simulink model "tf_rl_reward2"  (R2022a)
settings: Solver=VariableStepAuto  StartTime=0.0  StopTime=10.0  RelTol=1e-3
undefined symbols (not defined in the file or in its folder): DiscIntNeverNeededParam
libraries: simulink x3, rllib x1
settings Model: Creator=vicky  LastModifiedBy=archi

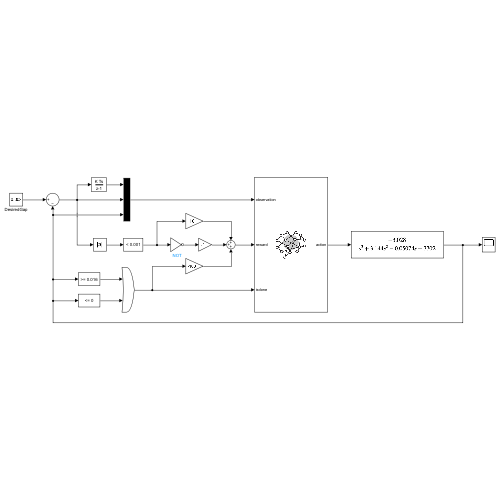
[thumbnail: Simulink's stored preview of the top-level diagram]
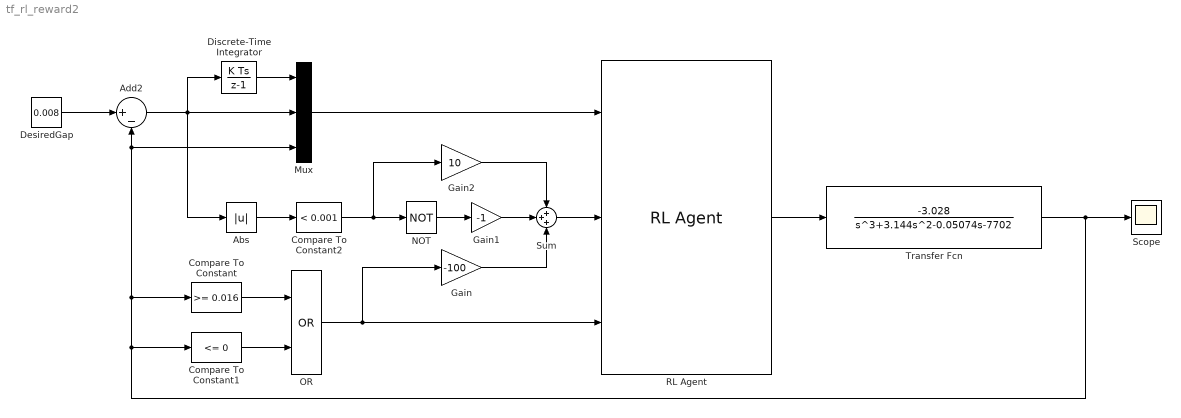
== system tf_rl_reward2 ==
  Abs : Abs  SaturateOnIntegerOverflow=off
  Add2 : Sum  Inputs=|+-
  Compare To Constant : simulink/Logic and Bit Operations/Compare To Constant  relop=>=  const=0.016  OutDataTypeStr=boolean
  Compare To Constant1 : simulink/Logic and Bit Operations/Compare To Constant  relop=<=  const=0  OutDataTypeStr=boolean
  Compare To Constant2 : simulink/Logic and Bit Operations/Compare To Constant  relop=<  const=0.001  OutDataTypeStr=boolean
  DesiredGap : Constant  Value=0.008
  Discrete-Time Integrator : DiscreteIntegrator  SampleTime=-1  ICPrevOutput=DiscIntNeverNeededParam  ICPrevScaledInput=DiscIntNeverNeededParam
  Gain : Gain  Gain=-100
  Gain1 : Gain  Gain=-1
  Gain2 : Gain  Gain=10
  Mux : Mux  Inputs=3
  NOT : Logic  Operator=NOT  IconShape=distinctive  AllPortsSameDT=off  OutDataTypeStr=boolean
  OR : Logic  Operator=OR  IconShape=distinctive  AllPortsSameDT=off  OutDataTypeStr=boolean
  RL Agent : rllib/RL Agent  Agent=rlDDPGAgent  ExternalActionAsInput=off  ProvideLastAction=off  ProvideCumRwd=off  TreatAsDirectFeedthrough=on  UseStrictObservationDataTypes=off
  Scope : Scope
  Sum : Sum  Inputs=+++
  Transfer Fcn : TransferFcn  Numerator=[-3.028]  Denominator=[1 3.144 -0.05074 -7702]
  wires:
  RL Agent/1 -> Transfer Fcn/1
  Add2/1 -> Mux/2, Abs/1, Discrete-Time Integrator/1
  Discrete-Time Integrator/1 -> Mux/1
  Mux/1 -> RL Agent/1
  DesiredGap/1 -> Add2/1
  Compare To Constant/1 -> OR/1
  Compare To Constant1/1 -> OR/2
  OR/1 -> Gain/1, RL Agent/3
  Transfer Fcn/1 -> Scope/1, Compare To Constant1/1, Compare To Constant/1, Mux/3, Add2/2
  Compare To Constant2/1 -> Gain2/1, NOT/1
  Abs/1 -> Compare To Constant2/1
  NOT/1 -> Gain1/1
  Gain/1 -> Sum/3
  Gain1/1 -> Sum/2
  Gain2/1 -> Sum/1
  Sum/1 -> RL Agent/2
